simulink model "Exercicio_7_Vinicius_Comparacao"  (R2018a)
settings: Solver=VariableStepAuto  StartTime=0.0  StopTime=40  RelTol=1e-3
undefined symbols (not defined in the file): AA, AAant, BB, BBant, DD, DDant, Eant, Fant, H, Hant, k2, KE, KF, KW, Ts, W
libraries: cstblocks x2
settings Model: Creator=vinic  LastModifiedBy=vinic

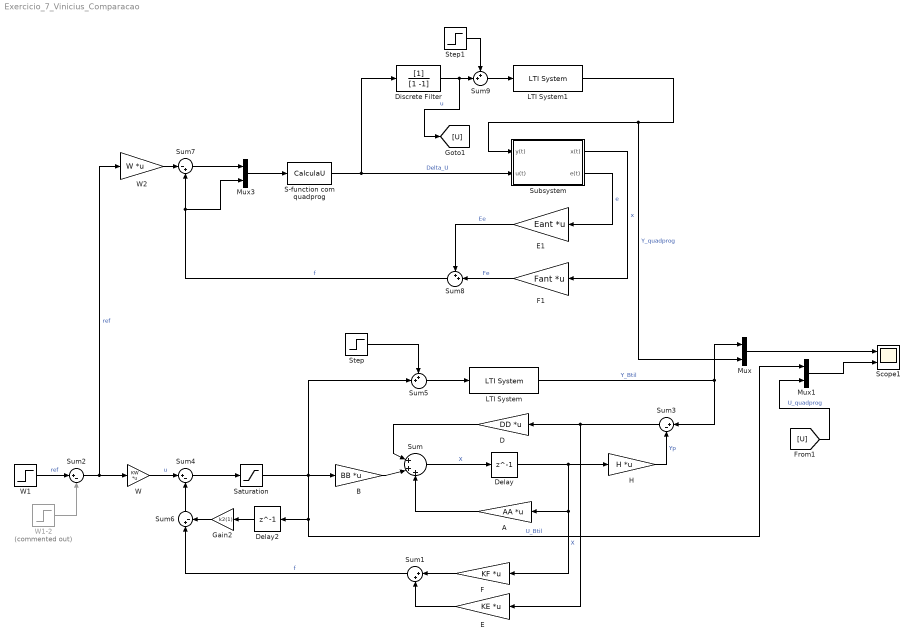
== system Exercicio_7_Vinicius_Comparacao ==
  A : Gain  Gain=AA  Multiplication=Matrix(K*u)
  B : Gain  Gain=BB  Multiplication=Matrix(K*u)
  D : Gain  Gain=DD  Multiplication=Matrix(K*u)
  Delay : Delay  DelayLength=1  SampleTime=Ts
  Delay2 : Delay  DelayLength=1
  Discrete Filter : DiscreteFilter  Denominator=[1 -1]  SampleTime=Ts
  E : Gain  Gain=KE  Multiplication=Matrix(K*u)
  E1 : Gain  Gain=Eant  Multiplication=Matrix(K*u)
  F : Gain  Gain=KF  Multiplication=Matrix(K*u)
  F1 : Gain  Gain=Fant  Multiplication=Matrix(K*u)
  Gain2 : Gain  Gain=k2(1)
  H : Gain  Gain=H  Multiplication=Matrix(K*u)
  LTI System : cstblocks/LTI System  sys=Processo  IC=[]
  LTI System1 : cstblocks/LTI System  sys=Processo  IC=[]
  Mux : Mux  Inputs=2
  Mux1 : Mux  Inputs=2
  Mux3 : Mux  Inputs=2
  S-function com quadprog : S-Function  FunctionName=CalculaU  Parameters=Parametros  SFunctionDeploymentMode=off  EnableBusSupport=off
  Saturation : Saturate  UpperLimit=0.3  LowerLimit=-0.2
  Scope1 : Scope  NumInputPorts=2
  Step : Step  Time=15  After=0.1  SampleTime=Ts
  Step1 : Step  Time=15  After=0.1  SampleTime=Ts
  Subsystem : Subsystem
  Sum : Sum  Inputs=|+++
  Sum1 : Sum  Inputs=|++
  Sum{2..4,6} (4 alike) : Sum  Inputs=|+-
  Sum5 : Sum  Inputs=++|
  Sum7 : Sum  Inputs=|-+
  Sum8 : Sum  Inputs=++|
  Sum9 : Sum  Inputs=++|
  W : Gain  Gain=KW  Multiplication=Matrix(K*u)
  W1 : Step  Time=0  SampleTime=Ts
  W1-2 : Step  Commented=on  Time=1.5  After=0.1  SampleTime=Ts
  W2 : Gain  Gain=W  Multiplication=Matrix(K*u)
  wires:
  Delay/1 -> F/1, A/1, H/1  "X"
  Sum8/1 -> Sum7/2, Mux3/2  "f"
  Delay2/1 -> Gain2/1
  Sum1/1 -> Sum6/1  "f"
  B/1 -> Sum/2
  Sum2/1 -> W2/1, W/1  "ref"
  S-function com quadprog/1 -> Discrete Filter/1, Subsystem/2(u(t))  "Delta_U"
  Sum3/1 -> E/1, D/1
  W2/1 -> Sum7/1
  E/1 -> Sum1/2
  Sum7/1 -> Mux3/1
  Discrete Filter/1 -> Sum9/2, [U]  "u"
  Subsystem/1(x(t)) -> F1/1  "x"
  D/1 -> Sum/1
  Subsystem/2(e(t)) -> E1/1  "e"
  [U] -> Mux1/2  "U_quadprog"
  Sum4/1 -> Saturation/1
  A/1 -> Sum/3
  Mux3/1 -> S-function com quadprog/1
  Mux1/1 -> Scope1/2
  Saturation/1 -> Mux1/1, Delay2/1, B/1, Sum5/2  "U_Btil"
  W1/1 -> Sum2/1  "ref"
  Mux/1 -> Scope1/1
  W/1 -> Sum4/1  "u"
  E1/1 -> Sum8/1  "Ee"
  Sum5/1 -> LTI System/1
  Sum6/1 -> Sum4/2
  LTI System/1 -> Mux/1, Sum3/1  "Y_Btil"
  Gain2/1 -> Sum6/2
  H/1 -> Sum3/2  "Yp"
  F1/1 -> Sum8/2  "Fe"
  W1-2/1 -> Sum2/2
  Step/1 -> Sum5/1
  F/1 -> Sum1/1
  Sum/1 -> Delay/1  "X"
  LTI System1/1 -> Mux/2, Subsystem/1(y(t))  "Y_quadprog"
  Sum9/1 -> LTI System1/1
  Step1/1 -> Sum9/1

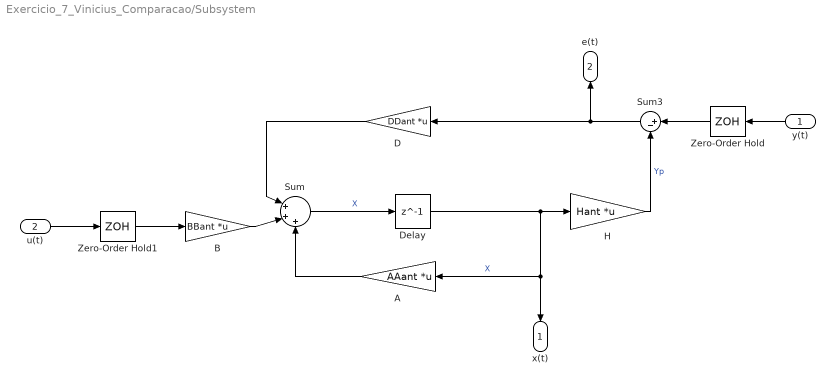
== system Exercicio_7_Vinicius_Comparacao/Subsystem ==
  y(t) : Inport
  u(t) : Inport  Port=2
  A : Gain  Gain=AAant  Multiplication=Matrix(K*u)
  B : Gain  Gain=BBant  Multiplication=Matrix(K*u)
  D : Gain  Gain=DDant  Multiplication=Matrix(K*u)
  Delay : Delay  DelayLength=1  SampleTime=Ts
  H : Gain  Gain=Hant  Multiplication=Matrix(K*u)
  Sum : Sum  Inputs=|+++
  Sum3 : Sum  Inputs=|+-
  Zero-Order Hold : ZeroOrderHold  SampleTime=Ts
  Zero-Order Hold1 : ZeroOrderHold  SampleTime=Ts
  x(t) : Outport
  e(t) : Outport  Port=2
  wires:
  y(t)/1 -> Zero-Order Hold/1
  u(t)/1 -> Zero-Order Hold1/1
  A/1 -> Sum/3
  B/1 -> Sum/2
  D/1 -> Sum/1
  Delay/1 -> x(t)/1, A/1, H/1  "X"
  Sum/1 -> Delay/1  "X"
  Zero-Order Hold1/1 -> B/1
  Zero-Order Hold/1 -> Sum3/1
  H/1 -> Sum3/2  "Yp"
  Sum3/1 -> D/1, e(t)/1
